simulink model "PIDTu4_34"  (Simulink 5.0)
settings: Solver=ode4  SolverMode=SingleTasking  StartTime=0.0  StopTime=10  FixedStep=0.1  RelTol=1e-3
settings Model: LastModifiedBy=ThinkPad

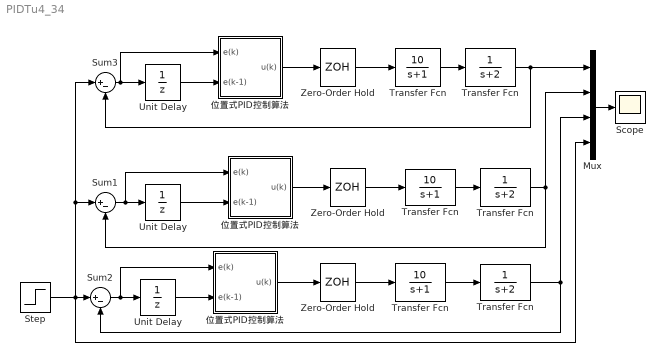
== system PIDTu4_34 ==
  " Transfer Fcn" : TransferFcn  Denominator=[1 2]
  " Transfer Fcn " : TransferFcn  Denominator=[1 2]
  " Transfer Fcn  " : TransferFcn  Numerator=[10]  Denominator=[1 1]
  " Unit Delay" : UnitDelay  SampleTime=0.1
  " Zero-Order Hold " : ZeroOrderHold  SampleTime=0.1
  " 位置式PID控制算法  " : Subsystem
  Mux : Mux
  Scope : Scope
      settings: YMin=0  YMax=1.6  SaveName=PIDtu_34  DataFormat=Array  MaxDataPoints=50000
  Step : Step  Time=0  SampleTime=0
  Sum1 : Sum  Inputs=|+-  SaturateOnIntegerOverflow=on
  Sum2 : Sum  Inputs=|+-  SaturateOnIntegerOverflow=on
  Sum3 : Sum  Inputs=|+-  SaturateOnIntegerOverflow=on
  Transfer Fcn : TransferFcn  Numerator=[10]  Denominator=[1 1]
  "Transfer Fcn " : TransferFcn  Denominator=[1 2]
  "Transfer Fcn  " : TransferFcn  Numerator=[10]  Denominator=[1 1]
  Unit Delay : UnitDelay  SampleTime=0.1
  "Unit Delay " : UnitDelay  SampleTime=0.1
  Zero-Order Hold : ZeroOrderHold  SampleTime=0.1
  "Zero-Order Hold " : ZeroOrderHold  SampleTime=0.1
  "位置式PID控制算法 " : Subsystem
  "位置式PID控制算法  " : Subsystem
  wires:
  Transfer Fcn/1 -> "Transfer Fcn "/1
  "位置式PID控制算法 "/1(u(k)) -> " Zero-Order Hold "/1
  " Zero-Order Hold "/1 -> Transfer Fcn/1
  "Transfer Fcn "/1 -> Mux/3, Sum2/2
  Step/1 -> Sum2/1, Sum3/1, Sum1/1, Mux/4
  Sum2/1 -> "位置式PID控制算法 "/1(e(k)), Unit Delay/1
  Unit Delay/1 -> "位置式PID控制算法 "/2(e(k-1))
  " Transfer Fcn  "/1 -> " Transfer Fcn "/1
  " 位置式PID控制算法  "/1(u(k)) -> "Zero-Order Hold "/1
  "Zero-Order Hold "/1 -> " Transfer Fcn  "/1
  " Transfer Fcn "/1 -> Sum1/2, Mux/2
  Sum1/1 -> " Unit Delay"/1, " 位置式PID控制算法  "/1(e(k))
  " Unit Delay"/1 -> " 位置式PID控制算法  "/2(e(k-1))
  "Transfer Fcn  "/1 -> " Transfer Fcn"/1
  "位置式PID控制算法  "/1(u(k)) -> Zero-Order Hold/1
  Zero-Order Hold/1 -> "Transfer Fcn  "/1
  " Transfer Fcn"/1 -> Sum3/2, Mux/1
  Sum3/1 -> "位置式PID控制算法  "/1(e(k)), "Unit Delay "/1
  "Unit Delay "/1 -> "位置式PID控制算法  "/2(e(k-1))
  Mux/1 -> Scope/1

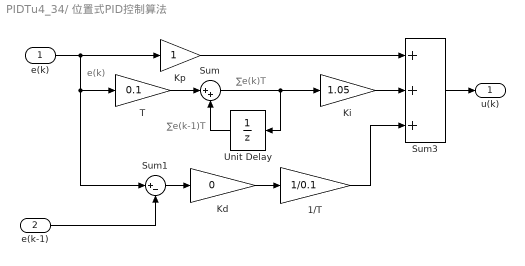
== system PIDTu4_34/ 位置式PID控制算法   ==
  note: ∑e(k-1)T
  note: ∑e(k)T
  note: e(k)
  e(k) : Inport
  e(k-1) : Inport  Port=2
  1/T : Gain  Gain=1/0.1  SaturateOnIntegerOverflow=on
  Kd : Gain  Gain=0  SaturateOnIntegerOverflow=on
  Ki : Gain  Gain=1.05  SaturateOnIntegerOverflow=on
  Kp : Gain  SaturateOnIntegerOverflow=on
  Sum : Sum  Inputs=|++  SaturateOnIntegerOverflow=on
  Sum1 : Sum  Inputs=|+-  SaturateOnIntegerOverflow=on
  Sum3 : Sum  Inputs=+++  SaturateOnIntegerOverflow=on
  T : Gain  Gain=0.1  SaturateOnIntegerOverflow=on
  Unit Delay : UnitDelay  Orientation=left  SampleTime=0.1
  u(k) : Outport
  wires:
  T/1 -> Sum/1
  e(k-1)/1 -> Sum1/2
  Unit Delay/1 -> Sum/2
  Sum/1 -> Ki/1, Unit Delay/1
  1/T/1 -> Sum3/3
  Kd/1 -> 1/T/1
  Sum3/1 -> u(k)/1
  Ki/1 -> Sum3/2
  Kp/1 -> Sum3/1
  e(k)/1 -> T/1, Sum1/1, Kp/1
  Sum1/1 -> Kd/1

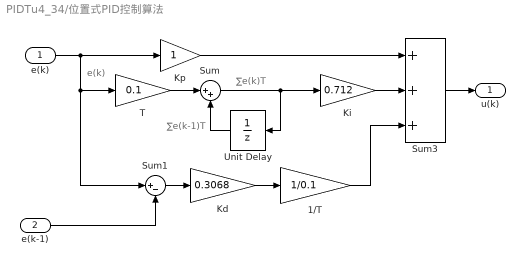
== system PIDTu4_34/位置式PID控制算法  ==
  note: e(k)
  note: ∑e(k)T
  note: ∑e(k-1)T
  e(k) : Inport
  e(k-1) : Inport  Port=2
  1/T : Gain  Gain=1/0.1  SaturateOnIntegerOverflow=on
  Kd : Gain  Gain=0.3068  SaturateOnIntegerOverflow=on
  Ki : Gain  Gain=0.712  SaturateOnIntegerOverflow=on
  Kp : Gain  SaturateOnIntegerOverflow=on
  Sum : Sum  Inputs=|++  SaturateOnIntegerOverflow=on
  Sum1 : Sum  Inputs=|+-  SaturateOnIntegerOverflow=on
  Sum3 : Sum  Inputs=+++  SaturateOnIntegerOverflow=on
  T : Gain  Gain=0.1  SaturateOnIntegerOverflow=on
  Unit Delay : UnitDelay  Orientation=left  SampleTime=0.1
  u(k) : Outport
  wires:
  Sum1/1 -> Kd/1
  e(k)/1 -> Kp/1, Sum1/1, T/1
  Kp/1 -> Sum3/1
  Ki/1 -> Sum3/2
  Sum3/1 -> u(k)/1
  Kd/1 -> 1/T/1
  1/T/1 -> Sum3/3
  Sum/1 -> Unit Delay/1, Ki/1
  Unit Delay/1 -> Sum/2
  e(k-1)/1 -> Sum1/2
  T/1 -> Sum/1

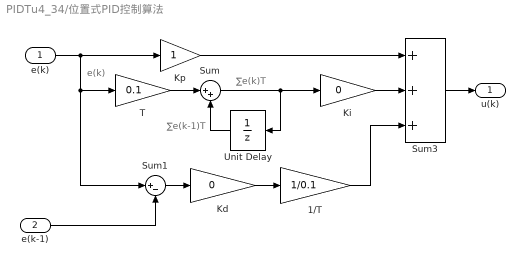
== system PIDTu4_34/位置式PID控制算法   ==
  note: e(k)
  note: ∑e(k)T
  note: ∑e(k-1)T
  e(k) : Inport
  e(k-1) : Inport  Port=2
  1/T : Gain  Gain=1/0.1  SaturateOnIntegerOverflow=on
  Kd : Gain  Gain=0  SaturateOnIntegerOverflow=on
  Ki : Gain  Gain=0  SaturateOnIntegerOverflow=on
  Kp : Gain  SaturateOnIntegerOverflow=on
  Sum : Sum  Inputs=|++  SaturateOnIntegerOverflow=on
  Sum1 : Sum  Inputs=|+-  SaturateOnIntegerOverflow=on
  Sum3 : Sum  Inputs=+++  SaturateOnIntegerOverflow=on
  T : Gain  Gain=0.1  SaturateOnIntegerOverflow=on
  Unit Delay : UnitDelay  Orientation=left  SampleTime=0.1
  u(k) : Outport
  wires:
  Sum1/1 -> Kd/1
  e(k)/1 -> Kp/1, Sum1/1, T/1
  Kp/1 -> Sum3/1
  Ki/1 -> Sum3/2
  Sum3/1 -> u(k)/1
  Kd/1 -> 1/T/1
  1/T/1 -> Sum3/3
  Sum/1 -> Unit Delay/1, Ki/1
  Unit Delay/1 -> Sum/2
  e(k-1)/1 -> Sum1/2
  T/1 -> Sum/1
